simulink model "AkkuSchrauber"  (R2025b)
settings: Solver=VariableStepAuto  StartTime=0.0  StopTime=10.0  RelTol=1e-3
settings Model: Creator=georg  LastModifiedBy=georg

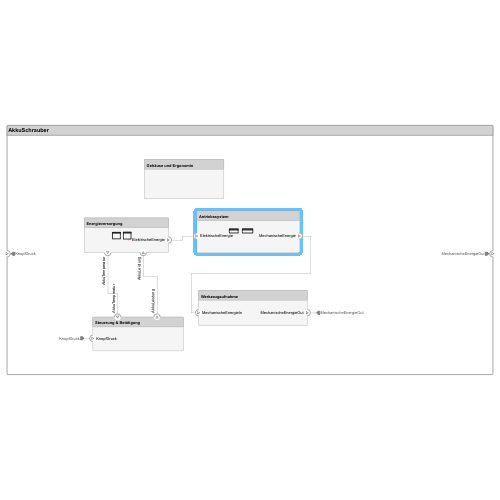
[thumbnail: Simulink's stored preview of the top-level diagram]
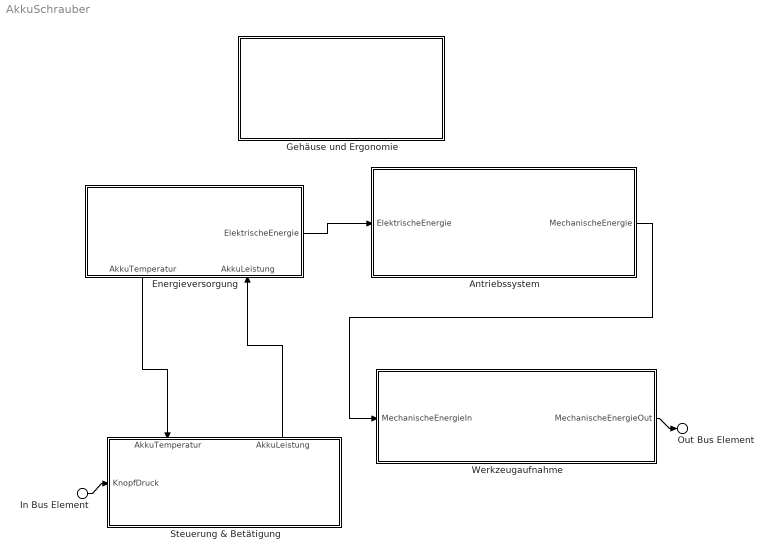
== system AkkuSchrauber ==
  In Bus Element : Inport  PortName=KnopfDruck
  Antriebssystem : Subsystem
      settings: PortSchema="{\"entries\":[{\"content\":{\"headerSize\":26,\"margin\":15,\"minimumSpacing\":25,\"sides\":[{\"content\":{\"connectorIds\":[\"In1\"]},\"type\":\"ConnectorPlacement.EquallySpacedRectSide\",\"uuid\":\"cc852fac-32eb-4011-bcf6-fcab5b2663da\"},{\"content\":{\"connectorIds\":[\"Out1\"],\"side\":\"RIGHT\"},\"type\":\"ConnectorPlacement.EquallySpacedRectSide\",\"uuid\":\"d3171f75-c9c1-4560-973d-d39e2a90e8f6\"},{\"content\":{\"side\":\"TOP\"},\"type\":\"ConnectorPlacement.EquallySpacedRectSide\",\"uuid\":\"092262db-a7ba-48ba-a662-ee6d84045f36\"},{\"content\":{\"side\":\"BOTTOM\"},\"type\":\"ConnectorPlacement.EquallySpacedRectSide\",\"uuid\":\"54dad4a2-5074-4fff-90f4-947ca757806d\"}]},\"type\":\"ConnectorPlacement.EquallySpacedConnector\",\"uuid\":\"cc59053b-a631-407b-8b33-4f9c5341cc4c\"}],\"packageUris\":[\"http://schema.mathworks.com/mf0/Connector/R2020b\"],\"version\":\"1.0\"}"
  Energieversorgung : Subsystem
      settings: PortSchema="{\"entries\":[{\"content\":{\"headerSize\":26,\"margin\":15,\"minimumSpacing\":25,\"sides\":[{\"content\":{},\"type\":\"ConnectorPlacement.EquallySpacedRectSide\",\"uuid\":\"cc852fac-32eb-4011-bcf6-fcab5b2663da\"},{\"content\":{\"connectorIds\":[\"Out2\"],\"side\":\"RIGHT\"},\"type\":\"ConnectorPlacement.EquallySpacedRectSide\",\"uuid\":\"d3171f75-c9c1-4560-973d-d39e2a90e8f6\"},{\"content\":{\"side\":\"TOP\"},\"type\":\"ConnectorPlacement.EquallySpacedRectSide\",\"uuid\":\"092262db-a7ba-48ba-a662-ee6d84045f36\"},{\"content\":{\"connectorIds\":[\"Out1\",\"In1\"],\"side\":\"BOTTOM\"},\"type\":\"ConnectorPlacement.EquallySpacedRectSide\",\"uuid\":\"d99f4f41-e8df-42d4-8e21-3abf6a0a8c93\"}]},\"type\":\"ConnectorPlacement.EquallySpacedConnector\",\"uuid\":\"cc59053b-a631-407b-8b33-4f9c5341cc4c\"}],\"packageUris\":[\"http://schema.mathworks.com/mf0/Connector/R2020b\"],\"version\":\"1.0\"}"
  Gehäuse und Ergonomie : Subsystem
      settings: PortSchema="{\"entries\":[{\"content\":{\"headerSize\":26,\"margin\":15,\"minimumSpacing\":25,\"sides\":[{\"content\":{},\"type\":\"ConnectorPlacement.EquallySpacedRectSide\",\"uuid\":\"cc852fac-32eb-4011-bcf6-fcab5b2663da\"},{\"content\":{\"side\":\"RIGHT\"},\"type\":\"ConnectorPlacement.EquallySpacedRectSide\",\"uuid\":\"d3171f75-c9c1-4560-973d-d39e2a90e8f6\"},{\"content\":{\"side\":\"TOP\"},\"type\":\"ConnectorPlacement.EquallySpacedRectSide\",\"uuid\":\"092262db-a7ba-48ba-a662-ee6d84045f36\"}]},\"type\":\"ConnectorPlacement.EquallySpacedConnector\",\"uuid\":\"cc59053b-a631-407b-8b33-4f9c5341cc4c\"}],\"packageUris\":[\"http://schema.mathworks.com/mf0/Connector/R2020b\"],\"version\":\"1.0\"}"
  Steuerung & Betätigung : Subsystem
      settings: PortSchema="{\"entries\":[{\"content\":{\"headerSize\":26,\"margin\":15,\"minimumSpacing\":25,\"sides\":[{\"content\":{\"connectorIds\":[\"In1\"]},\"type\":\"ConnectorPlacement.EquallySpacedRectSide\",\"uuid\":\"cc852fac-32eb-4011-bcf6-fcab5b2663da\"},{\"content\":{\"side\":\"RIGHT\"},\"type\":\"ConnectorPlacement.EquallySpacedRectSide\",\"uuid\":\"d3171f75-c9c1-4560-973d-d39e2a90e8f6\"},{\"content\":{\"connectorIds\":[\"In2\",\"Out1\"],\"side\":\"TOP\"},\"type\":\"ConnectorPlacement.EquallySpacedRectSide\",\"uuid\":\"092262db-a7ba-48ba-a662-ee6d84045f36\"},{\"content\":{\"side\":\"BOTTOM\"},\"type\":\"ConnectorPlacement.EquallySpacedRectSide\",\"uuid\":\"21120a4c-a7e8-4db0-b67b-affe915e66d4\"}]},\"type\":\"ConnectorPlacement.EquallySpacedConnector\",\"uuid\":\"cc59053b-a631-407b-8b33-4f9c5341cc4c\"}],\"packageUris\":[\"http://schema.mathworks.com/mf0/Connector/R2020b\"],\"version\":\"1.0\"}"
  Werkzeugaufnahme : Subsystem
      settings: PortSchema="{\"entries\":[{\"content\":{\"headerSize\":26,\"margin\":15,\"minimumSpacing\":25,\"sides\":[{\"content\":{\"connectorIds\":[\"In1\"]},\"type\":\"ConnectorPlacement.EquallySpacedRectSide\",\"uuid\":\"cc852fac-32eb-4011-bcf6-fcab5b2663da\"},{\"content\":{\"connectorIds\":[\"Out1\"],\"side\":\"RIGHT\"},\"type\":\"ConnectorPlacement.EquallySpacedRectSide\",\"uuid\":\"d3171f75-c9c1-4560-973d-d39e2a90e8f6\"},{\"content\":{\"side\":\"TOP\"},\"type\":\"ConnectorPlacement.EquallySpacedRectSide\",\"uuid\":\"092262db-a7ba-48ba-a662-ee6d84045f36\"}]},\"type\":\"ConnectorPlacement.EquallySpacedConnector\",\"uuid\":\"cc59053b-a631-407b-8b33-4f9c5341cc4c\"}],\"packageUris\":[\"http://schema.mathworks.com/mf0/Connector/R2020b\"],\"version\":\"1.0\"}"
  Out Bus Element : Outport  PortName=MechanischeEnergieOut
  wires:
  Energieversorgung/2(ElektrischeEnergie) -> Antriebssystem/1(ElektrischeEnergie)
  Energieversorgung/1(AkkuTemperatur) -> Steuerung & Betätigung/2(AkkuTemperatur)
  In Bus Element/1 -> Steuerung & Betätigung/1(KnopfDruck)
  Werkzeugaufnahme/1(MechanischeEnergieOut) -> Out Bus Element/1
  Antriebssystem/1(MechanischeEnergie) -> Werkzeugaufnahme/1(MechanischeEnergieIn)
  Steuerung & Betätigung/1(AkkuLeistung) -> Energieversorgung/1(AkkuLeistung)

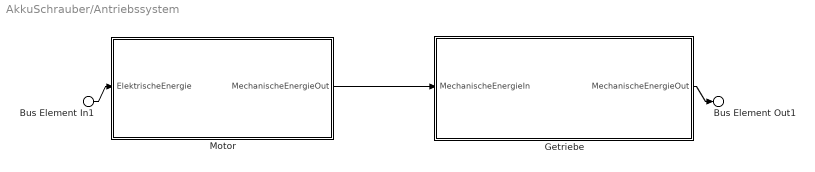
== system AkkuSchrauber/Antriebssystem ==
  Bus Element In1 : Inport  PortName=ElektrischeEnergie
  Getriebe : Subsystem
      settings: PortSchema="{\"entries\":[{\"content\":{\"headerSize\":26,\"margin\":15,\"minimumSpacing\":25,\"sides\":[{\"content\":{\"connectorIds\":[\"In1\"]},\"type\":\"ConnectorPlacement.EquallySpacedRectSide\",\"uuid\":\"cc852fac-32eb-4011-bcf6-fcab5b2663da\"},{\"content\":{\"connectorIds\":[\"Out1\"],\"side\":\"RIGHT\"},\"type\":\"ConnectorPlacement.EquallySpacedRectSide\",\"uuid\":\"d3171f75-c9c1-4560-973d-d39e2a90e8f6\"},{\"content\":{\"side\":\"TOP\"},\"type\":\"ConnectorPlacement.EquallySpacedRectSide\",\"uuid\":\"092262db-a7ba-48ba-a662-ee6d84045f36\"}]},\"type\":\"ConnectorPlacement.EquallySpacedConnector\",\"uuid\":\"cc59053b-a631-407b-8b33-4f9c5341cc4c\"}],\"packageUris\":[\"http://schema.mathworks.com/mf0/Connector/R2020b\"],\"version\":\"1.0\"}"
  Motor : Subsystem
      settings: PortSchema="{\"entries\":[{\"content\":{\"headerSize\":26,\"margin\":15,\"minimumSpacing\":25,\"sides\":[{\"content\":{\"connectorIds\":[\"In1\"]},\"type\":\"ConnectorPlacement.EquallySpacedRectSide\",\"uuid\":\"cc852fac-32eb-4011-bcf6-fcab5b2663da\"},{\"content\":{\"connectorIds\":[\"Out1\"],\"side\":\"RIGHT\"},\"type\":\"ConnectorPlacement.EquallySpacedRectSide\",\"uuid\":\"d3171f75-c9c1-4560-973d-d39e2a90e8f6\"},{\"content\":{\"side\":\"TOP\"},\"type\":\"ConnectorPlacement.EquallySpacedRectSide\",\"uuid\":\"092262db-a7ba-48ba-a662-ee6d84045f36\"}]},\"type\":\"ConnectorPlacement.EquallySpacedConnector\",\"uuid\":\"cc59053b-a631-407b-8b33-4f9c5341cc4c\"}],\"packageUris\":[\"http://schema.mathworks.com/mf0/Connector/R2020b\"],\"version\":\"1.0\"}"
  Bus Element Out1 : Outport  PortName=MechanischeEnergie
  wires:
  Bus Element In1/1 -> Motor/1(ElektrischeEnergie)
  Motor/1(MechanischeEnergieOut) -> Getriebe/1(MechanischeEnergieIn)
  Getriebe/1(MechanischeEnergieOut) -> Bus Element Out1/1

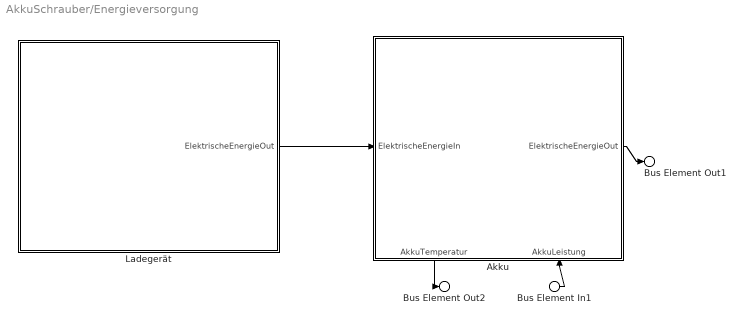
== system AkkuSchrauber/Energieversorgung ==
  Bus Element In1 : Inport  PortName=AkkuLeistung
  Akku : Subsystem
      settings: PortSchema="{\"entries\":[{\"content\":{\"headerSize\":26,\"margin\":15,\"minimumSpacing\":25,\"sides\":[{\"content\":{\"connectorIds\":[\"In2\"]},\"type\":\"ConnectorPlacement.EquallySpacedRectSide\",\"uuid\":\"cc852fac-32eb-4011-bcf6-fcab5b2663da\"},{\"content\":{\"connectorIds\":[\"Out2\"],\"side\":\"RIGHT\"},\"type\":\"ConnectorPlacement.EquallySpacedRectSide\",\"uuid\":\"d3171f75-c9c1-4560-973d-d39e2a90e8f6\"},{\"content\":{\"side\":\"TOP\"},\"type\":\"ConnectorPlacement.EquallySpacedRectSide\",\"uuid\":\"092262db-a7ba-48ba-a662-ee6d84045f36\"},{\"content\":{\"connectorIds\":[\"Out1\",\"In1\"],\"side\":\"BOTTOM\"},\"type\":\"ConnectorPlacement.EquallySpacedRectSide\",\"uuid\":\"7ef2578f-91d5-4674-ac0f-a81723ff669e\"}]},\"type\":\"ConnectorPlacement.EquallySpacedConnector\",\"uuid\":\"cc59053b-a631-407b-8b33-4f9c5341cc4c\"}],\"packageUris\":[\"http://schema.mathworks.com/mf0/Connector/R2020b\"],\"version\":\"1.0\"}"
  Ladegerät : Subsystem
      settings: PortSchema="{\"entries\":[{\"content\":{\"headerSize\":26,\"margin\":15,\"minimumSpacing\":25,\"sides\":[{\"content\":{},\"type\":\"ConnectorPlacement.EquallySpacedRectSide\",\"uuid\":\"cc852fac-32eb-4011-bcf6-fcab5b2663da\"},{\"content\":{\"connectorIds\":[\"Out1\"],\"side\":\"RIGHT\"},\"type\":\"ConnectorPlacement.EquallySpacedRectSide\",\"uuid\":\"d3171f75-c9c1-4560-973d-d39e2a90e8f6\"},{\"content\":{\"side\":\"TOP\"},\"type\":\"ConnectorPlacement.EquallySpacedRectSide\",\"uuid\":\"092262db-a7ba-48ba-a662-ee6d84045f36\"}]},\"type\":\"ConnectorPlacement.EquallySpacedConnector\",\"uuid\":\"cc59053b-a631-407b-8b33-4f9c5341cc4c\"}],\"packageUris\":[\"http://schema.mathworks.com/mf0/Connector/R2020b\"],\"version\":\"1.0\"}"
  Bus Element Out2 : Outport  PortName=AkkuTemperatur
  Bus Element Out1 : Outport  Port=2  PortName=ElektrischeEnergie
  wires:
  Ladegerät/1(ElektrischeEnergieOut) -> Akku/2(ElektrischeEnergieIn)
  Akku/2(ElektrischeEnergieOut) -> Bus Element Out1/1
  ? -> ?
  Akku/1(AkkuTemperatur) -> Bus Element Out2/1
  Bus Element In1/1 -> Akku/1(AkkuLeistung)

== system AkkuSchrauber/Gehäuse und Ergonomie ==

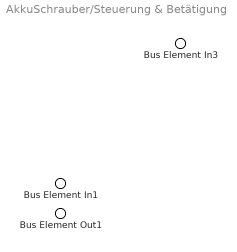
== system AkkuSchrauber/Steuerung & Betätigung ==
  Bus Element In3 : Inport  PortName=KnopfDruck
  Bus Element In1 : Inport  Port=2  PortName=AkkuTemperatur
  Bus Element Out1 : Outport  PortName=AkkuLeistung

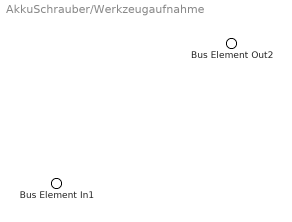
== system AkkuSchrauber/Werkzeugaufnahme ==
  Bus Element In1 : Inport  PortName=MechanischeEnergieIn
  Bus Element Out2 : Outport  PortName=MechanischeEnergieOut

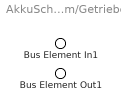
== system AkkuSchrauber/Antriebssystem/Getriebe ==
  Bus Element In1 : Inport  PortName=MechanischeEnergieIn
  Bus Element Out1 : Outport  PortName=MechanischeEnergieOut

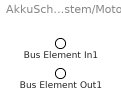
== system AkkuSchrauber/Antriebssystem/Motor ==
  Bus Element In1 : Inport  PortName=ElektrischeEnergie
  Bus Element Out1 : Outport  PortName=MechanischeEnergieOut

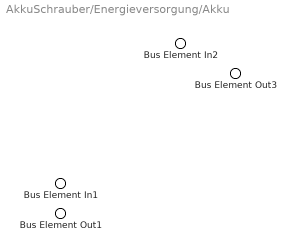
== system AkkuSchrauber/Energieversorgung/Akku ==
  Bus Element In2 : Inport  PortName=AkkuLeistung
  Bus Element In1 : Inport  Port=2  PortName=ElektrischeEnergieIn
  Bus Element Out3 : Outport  PortName=AkkuTemperatur
  Bus Element Out1 : Outport  Port=2  PortName=ElektrischeEnergieOut

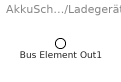
== system AkkuSchrauber/Energieversorgung/Ladegerät ==
  Bus Element Out1 : Outport  PortName=ElektrischeEnergieOut
